simulink model "SIM_6DOF"  (R2025b)
settings: Solver=VariableStepAuto  StartTime=0.0  StopTime=120  RelTol=1e-3
libraries: aerolibfltsims x2, aerolibpropulsion2 x1
settings Model: Creator=papar  LastModifiedBy=papar

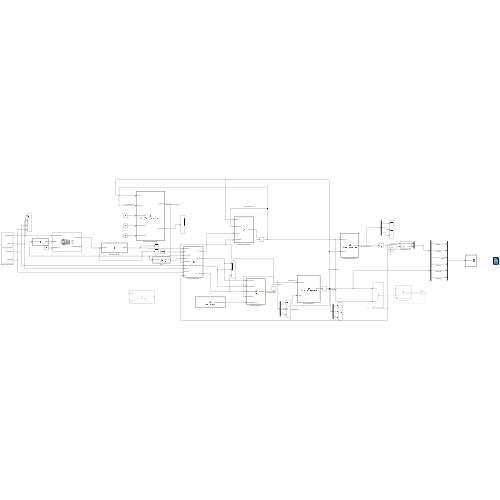
[thumbnail: Simulink's stored preview of the top-level diagram]
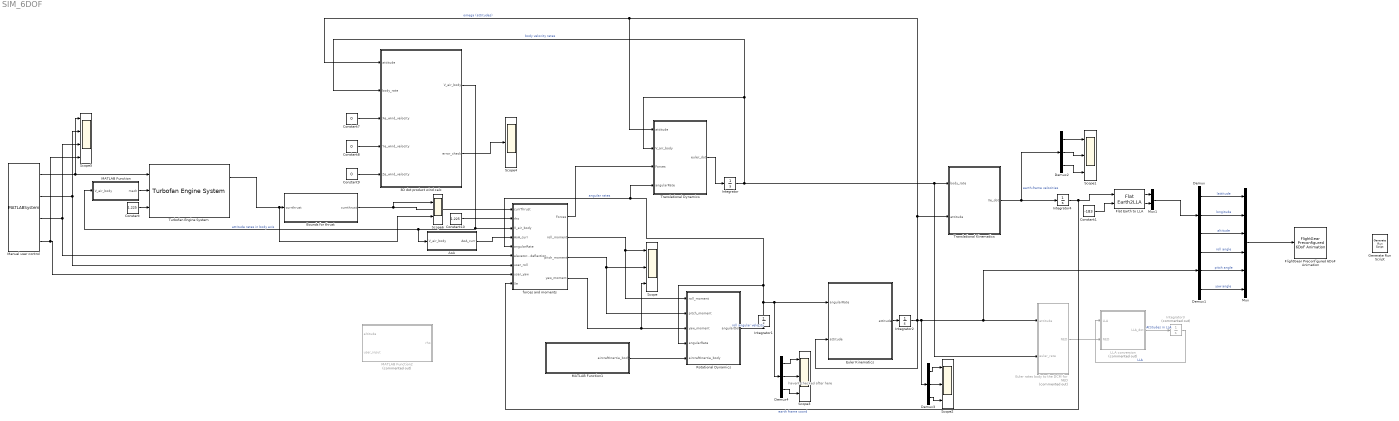
== system SIM_6DOF ==
  note: havent checked after here
  3D dot product wind calc : MATLAB Function  TreatAsAtomicUnit=on
  AoA : MATLAB Function  TreatAsAtomicUnit=on
  Bounds for thrust : MATLAB Function  TreatAsAtomicUnit=on
  Constant : Constant  Value=1.225
  Constant1 : Constant  Value=-183
  Constant10 : Constant  Value=1.225
  Constant7 : Constant  Value=0
  Constant8 : Constant  Value=0
  Constant9 : Constant  Value=0
  Demux{,1..4} (5 alike) : Demux  Outputs=3
  Euler Kinematics : MATLAB Function  TreatAsAtomicUnit=on
  Euler rates body to the DCM for NED : MATLAB Function  Commented=on  TreatAsAtomicUnit=on
  Flat Earth to LLA : FlatEarth2LLA
  FlightGear Preconfigured 6DoF Animation : aerolibfltsims/FlightGear Preconfigured 6DoF Animation  xFlightGearVersion=v2019.1  DestinationIpAddress=127.0.0.1  DestinationPort=5502  SampleTime=1/30  packetVersion=24
  Generate Run Script : aerolibfltsims/Generate Run Script  Architecture=Win64  dataFlow=Send  GeometryModelName=c172p  AirportId=KSEA  RunwayId=34R  InitialAltitude=0  InitialHeading=0  OffsetDistance=0  OffsetAzimuth=0  InstallScenery=off  DisableShaders=on  OriginAddress=127.0.0.1  DestinationPort=5502  OriginPort=5505  LocalAddress=127.0.0.1  OutputFileName=runfg.bat  FlightGearBaseDirectory=C:\Program Files\FlightGear 2024.1
  Integrator{,1..2,4} (4 alike) : Integrator
  Integrator3 : Integrator  Commented=on
  LLA conversion : MATLAB Function  Commented=on  TreatAsAtomicUnit=on
  MATLAB Function : MATLAB Function  TreatAsAtomicUnit=on
  MATLAB Function1 : MATLAB Function  TreatAsAtomicUnit=on
  MATLAB Function2 : MATLAB Function  Commented=on  TreatAsAtomicUnit=on
  Manual user control : MATLABSystem  System=user_key_inputs  throttle_rate=0.5  init_throttle=0  user_control_block_update=0.01
      mask Type: user_key_inputs
  Mux : Mux  Inputs=6
  Mux1 : Mux  Inputs=2
  Rotational Dynamics : MATLAB Function  TreatAsAtomicUnit=on
  Scope{,1..3} (4 alike) : Scope  NumInputPorts=3
      Scope settings: ActiveDisplayYMinimum=-4.728663837625831  ActiveDisplayYMaximum=4.4335666022021805
      Scope1 settings: ActiveDisplayYMinimum=-4.93510226383194  ActiveDisplayYMaximum=5.6713247490739631
      Scope2 settings: ActiveDisplayYMinimum=-4.9456036767160052  ActiveDisplayYMaximum=6.1911446868351954  DataLoggingVariableName=ScopeData2
      Scope3 settings: ActiveDisplayYMinimum=-4.9456036767160052  ActiveDisplayYMaximum=6.1911446868351954  DataLoggingVariableName=ScopeData3
  Scope4 : Scope
      settings: ActiveDisplayYMinimum=-5.40759459482811  ActiveDisplayYMaximum=5.1988324180777932  DataLoggingVariableName=ScopeData4
  Scope5 : Scope  NumInputPorts=4
      settings: ActiveDisplayYMinimum=-0.30490675026958991  ActiveDisplayYMaximum=1.9451086406647558  DataLoggingVariableName=ScopeData5
  Scope6 : Scope  NumInputPorts=2
      settings: ActiveDisplayYMinimum=-5061.7647583692151  ActiveDisplayYMaximum=45555.882825322944  DataLoggingVariableName=ScopeData6
  Translational Dynamics : MATLAB Function  TreatAsAtomicUnit=on
  Translational Kinematics : MATLAB Function  TreatAsAtomicUnit=on
  Turbofan Engine System : aerolibpropulsion2/Turbofan Engine System  units=Metric (MKS)  ic_source=Internal  IC=0  Fmax=45000  tau=1  SFC=0.35  Nt=0.9
  forces and moments : MATLAB Function  TreatAsAtomicUnit=on
  wires:
  Translational Kinematics/1(Xe_dot) -> Demux2/1, Integrator4/1  "earth-frame velocities"
  Mux/1 -> FlightGear Preconfigured 6DoF Animation/1
  Demux/1 -> Mux/1  "lattitude"
  Demux/2 -> Mux/2  "longitude"
  Demux/3 -> Mux/3  "altitude"
  Demux1/1 -> Mux/4  "roll angle"
  Demux1/2 -> Mux/5  "pitch angle"
  Demux1/3 -> Mux/6  "yaw angle"
  LLA conversion/1(LLA_dot) -> Integrator3/1  "Attitudes in LLA"
  3D dot product wind calc/1(V_air_body) -> forces and moments/3(V_air_body), AoA/1(V_air_body), MATLAB Function/1(V_air_body)  "attitude rates in body axis"
  Manual user control/1 -> Scope5/1, Turbofan Engine System/1
  MATLAB Function/1(mach) -> Turbofan Engine System/2
  Rotational Dynamics/1(angularDot) -> Integrator1/1  "roll angular velocity"
  Manual user control/2 -> Scope5/2, forces and moments/7(user_roll)
  Constant/1 -> Turbofan Engine System/3
  Constant7/1 -> 3D dot product wind calc/3(Xe_wind_velocity)
  Constant9/1 -> 3D dot product wind calc/5(Ze_wind_velocity)
  Constant8/1 -> 3D dot product wind calc/4(Ye_wind_velocity)
  Constant10/1 -> forces and moments/2(rho)
  forces and moments/1(Forces) -> Translational Dynamics/3(Forces)
  forces and moments/2(roll_moment) -> Scope/1, Rotational Dynamics/1(roll_moment)
  forces and moments/3(pitch_moment) -> Scope/2, Rotational Dynamics/2(pitch_moment)
  forces and moments/4(yaw_moment) -> Scope/3, Rotational Dynamics/3(yaw_moment)
  MATLAB Function1/1(aircraftInertia_body) -> Rotational Dynamics/5(aircraftInertia_body)
  Integrator/1 -> Translational Dynamics/2(V_air_body), 3D dot product wind calc/2(body_rate), Euler rates body to the DCM for NED/2(euler_rate), Translational Kinematics/1(body_rate)  "body velocity rates"
  Euler rates body to the DCM for NED/1(NED) -> LLA conversion/2(NED)
  Translational Dynamics/1(euler_dot) -> Integrator/1
  Integrator1/1 -> Rotational Dynamics/4(angularRate), Translational Dynamics/4(angularRate), forces and moments/5(angularRate), Demux4/1, Euler Kinematics/1(angularRate)  "angular rates"
  Integrator2/1 -> Translational Kinematics/2(attitude), Translational Dynamics/1(attitude), 3D dot product wind calc/1(attitude), Demux3/1, Demux1/1, Euler rates body to the DCM for NED/1(attitude), Euler Kinematics/2("attitude ")  "omega (attitudes)"
  Manual user control/3 -> Scope5/3, forces and moments/6(elevator_deflection)
  Euler Kinematics/1(attitude) -> Integrator2/1
  Integrator3/1 -> LLA conversion/1(LLA)  "LLA"
  Integrator4/1 -> forces and moments/9(Xe), Flat Earth to LLA/1  "earth frame coord"
  AoA/1(AoA_curr) -> forces and moments/4(AoA_curr)
  Mux1/1 -> Demux/1
  Flat Earth to LLA/1 -> Mux1/1
  Flat Earth to LLA/2 -> Mux1/2
  Constant1/1 -> Flat Earth to LLA/2
  Turbofan Engine System/1 -> Scope6/2, Bounds for thrust/1("currthrust ")
  Demux2/1 -> Scope1/1
  Demux2/2 -> Scope1/2
  Demux2/3 -> Scope1/3
  Demux3/1 -> Scope2/1
  Demux3/2 -> Scope2/2
  Demux3/3 -> Scope2/3
  Demux4/1 -> Scope3/1
  Demux4/2 -> Scope3/2
  Demux4/3 -> Scope3/3
  Bounds for thrust/1(currthrust) -> Scope6/1, forces and moments/1(currThrust)
  Manual user control/4 -> Scope5/4, forces and moments/8(user_yaw)
  3D dot product wind calc/2(error_check) -> Scope4/1

== matlab function SIM_6DOF/MATLAB Function ==
  data: V_air_body input double size=[3 1]; mach output
function mach = fcn(V_air_body)

%setting var
soundVelocity = 340.3;

%magnitude of body axis velocity
    %sub var
u_wind = V_air_body(1);
v_wind = V_air_body(2);
w_wind = V_air_body(3);

%/*calcualte the magnitude of the body axis velcoity from
%the effect of wind*\
mag_Vel_Body = sqrt(u_wind.^2 + v_wind.^2 + w_wind.^2);

%calcuate mach
mach = mag_Vel_Body ./ soundVelocity;

== matlab function SIM_6DOF/MATLAB Function1 ==
  data: aircraftInertia_body output; user_input parameter
function aircraftInertia_body = calculate_inertia(user_input)

%Estimating X CG
XCG = sum(user_input.massArray .* user_input.xArray) ./ user_input.total_mass;

component_x_from_CG = user_input.xArray - XCG;

%Calculation of each inertia
x_inertia = 1000;

y_inertia = sum(user_input.massArray .* component_x_from_CG.^2);

z_inertia = sum(user_input.massArray .* component_x_from_CG.^2);

%Building a simple matrix oif the inertias
aircraftInertia_body = diag([x_inertia y_inertia z_inertia]);

== matlab function SIM_6DOF/LLA conversion ==
  data: LLA_dot output double size=[3 1]; LLA input double size=[3 1]; NED input double size=[3 1]
function LLA_dot = LLA_conversion(LLA,NED)

%set var
northVelocity = NED(1);
eastVelocity = NED(2);
downVelocity = NED(3);

lat = LLA(1); 
altitude = LLA(3); 

%Setting our variables
radius_prime_vertical = 1;
lat_dot = northVelocity ./  + altitude;

lon_dot = eastVelocity ./ (radius_prime_vertical + altitude) .* cos(lat);

altitude_dot = -downVelocity;

LLA_dot = [lat_dot; lon_dot; altitude_dot];

== matlab function SIM_6DOF/Euler rates body to the DCM for NED ==
  data: attitude input; euler_rate input; NED output
function NED = fcn(attitude,euler_rate)

phi = attitude(1);
theta = attitude(2);
psi = attitude(3);

u = euler_rate(1);
v = euler_rate(2);
w = euler_rate(3);

V_N = cos(theta) .* cos(psi) .* u + (sin(phi) .* sin(theta) .* cos(psi) -...
    cos(phi) .* sin(psi)) .* v + (cos(phi) .* sin(theta) .* cos(psi) + ...
    sin(phi) .* sin(psi)) .* w;

V_E = cos(theta) .* sin(psi) .* u + (sin(phi) .* sin(theta) .* sin(psi) +...
    cos(phi) .* cos(psi)) .* v + (cos(phi) .* sin(theta) .* sin(psi) - ...
    sin(phi) .* cos(psi)) .* w;

V_D = -sin(theta) .* u + sin(phi) .* cos(theta) .* v +...
    cos(phi) .* cos(theta) .* w;

NED = [V_N, V_E, V_D];

== matlab function SIM_6DOF/MATLAB Function2 ==
  data: altitude input; rho output; user_input input
function rho = altitude_find_rho(altitude,user_input)
rho_SL = 1.225;
temp_SL = 288.15;
temp_lapse_rate = 0.0065;
air_gas = 287.05;

rho = rho_SL .* (1 - (temp_lapse_rate .* altitude) ./ temp_SL).^ ...
    ((user_input.Gravity ./ (air_gas .* temp_lapse_rate)) - 1);

== matlab function SIM_6DOF/AoA ==
  data: V_air_body input; AoA_curr output
function AoA_curr = calculate_AoA(V_air_body)

%set var
u_air_body = V_air_body(1);
w_air_body = V_air_body(3);

AoA_curr = atan2(w_air_body, u_air_body);

== matlab function SIM_6DOF/Translational Dynamics ==
  data: attitude input double size=[3 1]; V_air_body input double size=[3 1]; Forces input double size=[3 1]; angularRate input double size=[3 1]; euler_dot output double size=[3 1]; user_input parameter
function euler_dot = fcn(attitude, V_air_body, Forces, angularRate, user_input)

%setting var
p = angularRate(1);
q = angularRate(2);
r = angularRate(3);

phi = attitude(1);
theta = attitude(2);

Fx = Forces(1);
Fy = Forces(2);
Fz = Forces(3);

%sub formula

u_air_body = V_air_body(1);
v_air_body = V_air_body(2);
w_air_body = V_air_body(3);

% AoA_curr = atan2(w_air_body, u_air_body);
%mass
mass_TO = user_input.total_mass;

%accleration the rate of change of u, v, and w
u_dot = r .* v_air_body - q .* w_air_body + Fx ./ mass_TO - ...
    user_input.Gravity .* sin(theta);

v_dot =  p .* w_air_body - r .* u_air_body + Fy ./ mass_TO + ...
    user_input.Gravity .* sin(phi) .* cos(theta);

w_dot = q * u_air_body - p .* v_air_body + Fz ./ mass_TO + ...
    user_input.Gravity .* cos(phi) .* cos(theta);

%acceleration of aircraft relative to wind

euler_dot = [u_dot;v_dot;w_dot];

== matlab function SIM_6DOF/forces and moments ==
  data: currThrust input double size=[1 1]; Forces output double size=[3 1]; rho input double size=[1 1]; roll_moment output double size=[1 1]; pitch_moment output double size=[1 1]; yaw_moment output double size=[1 1]; V_air_body input double size=[3 1]; AoA_curr input double size=[1 1]; angularRate input double size=[3 1]; elevator_deflection input double size=[1 1]; user_roll input double size=[1 1]; user_yaw input double size=[1 1]; user_input parameter; Xe input size=[3 1]
function [Forces,roll_moment,pitch_moment,yaw_moment] = fcn(currThrust, rho, V_air_body, AoA_curr, angularRate, ...
    elevator_deflection, user_roll, user_yaw, user_input, Xe) % Add phi and theta later

q = angularRate(2);

Ze = Xe(3);

V_air = norm(V_air_body);

%use of functions and arrays
AoA_curr_array = rad2deg(AoA_curr);
elevator_deflection_deg = rad2deg(elevator_deflection);

C_L_AoA = interp1(user_input.AoA_array, ...
    user_input.C_L_AoA_array, AoA_curr_array, "linear", "extrap");

C_D_AoA = interp1(user_input.AoA_array, ...
    user_input.C_D_AoA_array, AoA_curr_array, "linear", "extrap");

delta_C_M_elevator = interp1(user_input.elevator_deflection_array, ...
    user_input.delta_C_m_elevator_array, elevator_deflection_deg, "linear", ...
    "extrap");

%sub formulas HERE

%pitch rate nondimensional
if V_air < 1e-8
    pitch_rate = 0;
else
    pitch_rate = q .* user_input.MAC_ref ./ (2 .* V_air);
end


    %Current pitching moment coeff
C_M_curr = user_input.C_M0 + user_input.C_m_AoA_derivative .* AoA_curr ...
    + user_input.C_m_q .* pitch_rate + delta_C_M_elevator;


    %dynamic pressure
dynamicPressure = 0.5 * rho .* V_air.^2;

%Lift and drag in body axis
liftBody = dynamicPressure .* user_input.Wing_area .* C_L_AoA;

dragBody = dynamicPressure .* user_input.Wing_area .* C_D_AoA;

%The forces
Fx = currThrust - dragBody .* cos(AoA_curr) + liftBody .* sin(AoA_curr);

Fy = 0;

Fz = -dragBody .* sin(AoA_curr) - liftBody .* cos(AoA_curr);

Forces = [Fx;0;Fz];

if Ze >= 0
    normalFz = user_input.total_mass * user_input.Gravity;
else
    normalFz = 0;
end

Forces = Forces + [0; 0; -normalFz];

%
roll_moment = user_roll;

% The pitching moment
 pitch_moment = dynamicPressure .* user_input.Wing_area .* user_input.MAC_ref .* C_M_curr;


yaw_moment = user_yaw;

== matlab function SIM_6DOF/Rotational Dynamics ==
  data: roll_moment input size=[1 1]; angularDot output double size=[3 1]; pitch_moment input size=[1 1]; yaw_moment input size=[1 1]; angularRate input size=[3 1]; aircraftInertia_body input size=[3 3]
function angularDot = fcn(roll_moment, pitch_moment, yaw_moment, angularRate, aircraftInertia_body)

p = angularRate(1);
q = angularRate(2);
r = angularRate(3);

angularRate = [p;q;r];

%/*moment as a vector*\
moment_vector = [roll_moment; pitch_moment; yaw_moment];

%Rotational dynamics

%Remember that the "\" this is matlab way of solving for matrix eqn
angularDot = aircraftInertia_body \ (moment_vector - cross(angularRate, ...
    aircraftInertia_body * angularRate));

== matlab function SIM_6DOF/Euler Kinematics ==
  data: angularRate input; attitude input; attitude output
function attitude = calculate_eulerKinematics(angularRate,attitude)

phi = attitude(1);
theta = attitude(2);

%Settign vairables
p = angularRate(1);
q = angularRate(2);
r = angularRate(3);

%Euler kinematics
phi_dot = p + q .* sin(phi) .* tan(theta) + r .* cos(phi) .* tan(theta);

theta_dot = q .* cos(phi) - r .* sin(phi);

psi_dot = q .* sin(phi) ./ cos(theta) + r .* cos(phi) ./ cos(theta);

attitude = [phi_dot; theta_dot; psi_dot];

== matlab function SIM_6DOF/Translational Kinematics ==
  data: body_rate input; attitude input; Xe_dot output
function Xe_dot   = calculate_positionRate(body_rate,attitude)

phi = attitude(1);
theta = attitude(2);
psi = attitude(3);

u = body_rate(1);
v = body_rate(2);
w = body_rate(3);

x_dot = cos(theta) .* cos(psi) .* u + (sin(phi) .* sin(theta) .* cos(psi) -...
    cos(phi) .* sin(psi)) .* v + (cos(phi) .* sin(theta) .* cos(psi) + ...
    sin(phi) .* sin(psi)) .* w;

y_dot = cos(theta) .* sin(psi) .* u + (sin(phi) .* sin(theta) .* sin(psi) + ...
    cos(phi) .* cos(psi)) .* v + (cos(phi) .* sin(theta) .* sin(psi) - ...
    sin(phi) .* cos(psi)) .* w;

z_dot = -sin(theta) .* u + sin(phi) .* cos(theta) .* v + cos(phi) .* ...
    cos(theta) .* w;

Xe_dot = [x_dot; y_dot; z_dot];

== matlab function SIM_6DOF/3D dot product wind calc ==
  data: attitude input; body_rate input; V_air_body output double size=[3 1]; Xe_wind_velocity input; Ye_wind_velocity input; Ze_wind_velocity input; error_check output
function [V_air_body,error_check]  = find_aircraft_relative_to_wind_velocity(attitude, ...
    body_rate, Xe_wind_velocity, Ye_wind_velocity, Ze_wind_velocity)

%u, v, and w represents the aircraft velocity in body axis. So the u, v, w
%with wind means the velocity of the aircraft relative to wind.

%We are expressing components with Xe, Ye, and Ze if in earth frame coord.
%If body axis is being expressed in earth coord we note both the names and
% use context to understand its true coord.*\

%setting variables
u = body_rate(1);
v = body_rate(2);
w = body_rate(3);

phi = attitude(1);
theta = attitude(2);
psi = attitude(3);

%trig values in radians

phi_cos = cos(phi);

phi_sin = sin(phi);

theta_cos = cos(theta);

theta_sin = sin(theta);

psi_cos = cos(psi);

psi_sin = sin(psi);




%/*The body axis of aircraft as a unit vector in earth coord. However this is not
%the same as earth frame coord. We are only expressing the body axis in
%earth coord as a unit vector.*\

aircraft_x_body_earth = [theta_cos .* psi_cos; theta_cos .* psi_sin; -theta_sin];

aircraft_y_body_earth = [theta_sin .* phi_sin .* psi_cos - phi_cos .* psi_sin; phi_sin .* ...
    theta_sin .* psi_sin + phi_cos .* psi_cos; phi_sin .* theta_cos];

aircraft_z_body_earth = [phi_cos .* theta_sin .* psi_cos + phi_sin .* psi_sin; ...
    phi_cos .* theta_sin .* psi_sin - phi_sin .* psi_cos; ...
    phi_cos .* theta_cos];



% /*Users need to input wind as earth frame components when asked in
% setup. Storing the vectors into earth frame coordinates*\

e_wind = [Xe_wind_velocity; Ye_wind_velocity; Ze_wind_velocity];

%/*We stored wind velocity earth coord in function to then do dot product in 3D. We
% expressed the aircraft body axis in earth coord for the wind coord in
% earth frames. By doing the dot product we find how the wind reacts along
% the aircraft. Thus results in body axis.*\

Xb_wind_velocity = dot(e_wind, aircraft_x_body_earth);

Yb_wind_velocity = dot(e_wind, aircraft_y_body_earth);

Zb_wind_velocity = dot(e_wind, aircraft_z_body_earth);


% Now subtract wind velocity in body axis from the normal aircraft velocity
% body axis, to get the aircrafts velocity that is relative to the air. For
% example, this says the aircraft moving from the surrounding air so if
% wind is -2 m/s, that is increasing the velocity.

u_relative_air = u - Xb_wind_velocity;

v_relative_air = v - Yb_wind_velocity;

w_relative_air = w - Zb_wind_velocity;

V_air_body = [u_relative_air; v_relative_air; w_relative_air];

error_check = V_air_body - body_rate;
%output as a single vector
end

== matlab function SIM_6DOF/Bounds for thrust ==
  data: currthrust input; currthrust output; user_input parameter
function currthrust = fcn(currthrust,user_input)

if (currthrust >= user_input.thrust)

    currthrust = max(currthrust, user_input.thrust);

end
